simulink model "rov_kinematics_level2"  (R2024b)
settings: Solver=FixedStepAuto  StartTime=0.0  StopTime=90  FixedStep=0.01  RelTol=1e-3
values from neighbouring files (symbols this model uses):
  A = A0    [buildGainGrid.m]    (also in rovHoverModel.m = [ zeros(6),       eye(6))
  B = B0    [buildGainGrid.m]    (also in makeFeedForwardTau.m = p.rho * p.g * p.volume; rovHoverModel.m = [ zeros(6))
  C_integration = C(1:6,:)    [main_hover_controller.m]
  C_real = C_full(meas_idx,:)    [main_hover_controller.m]
  D = diag(p.D_lin) + diag(p.D_quad .* abs(nu))    [computeDynamicsSimple.m]    (also in makeFeedForwardTau.m = D_lin + D_quad; rovHoverModel.m = zeros(12,6))
  Ki = Kfull(:, n+1:end)    [designHoverController.m]    (also in designHoverControllerAtTrim.m)
  L = 0.5    [animateTrajectoryGIF.m]    (also in buildMixingMatrix.m = 0.575; main_hover_controller.m = lqe(A, G, C_real, Qn, Rn); test_linear_hover.m = 400; visualizeTrajectory.m = 1)
undefined symbols (not defined in the file or in its folder): schedData
settings Model: Creator=eirikvarnes  LastModifiedBy=eirikvarnes
settings DataIOCC: SaveFormat=Array  SaveTime=off  ReturnWorkspaceOutputs=off  OutputSaveName=eta

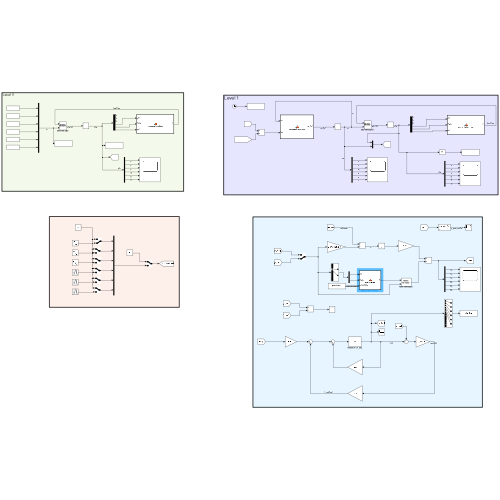
[thumbnail: Simulink's stored preview of the top-level diagram]
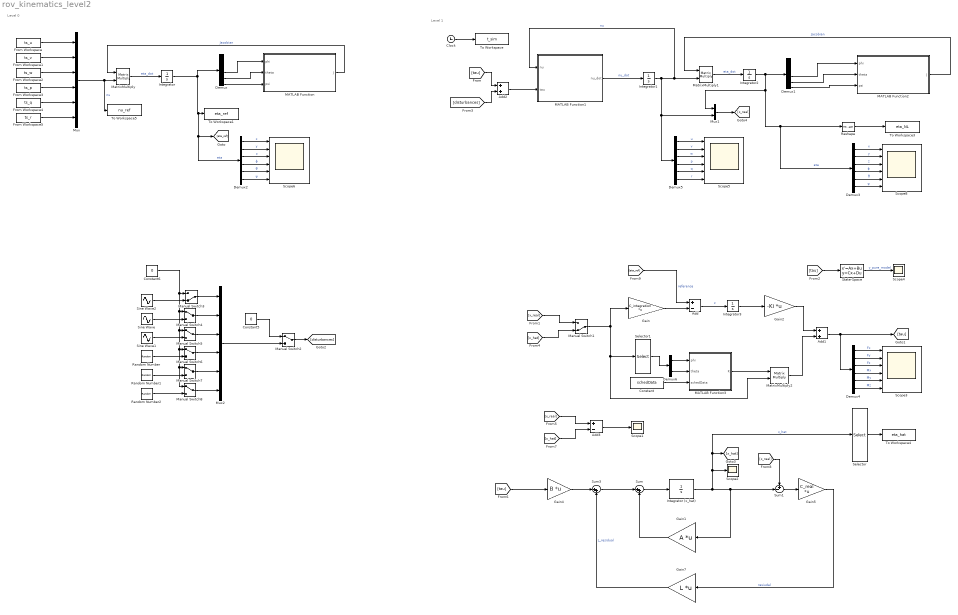
== system rov_kinematics_level2 ==
  note: Level 1
  note: Level 0
  Add : Sum  Inputs=+-
  Add1 : Sum
  Add2 : Sum
  Add3 : Sum  Inputs=+-
  Clock : Clock
  Constant : Constant  Value=schedData  OutDataTypeStr=Bus: schedDataBus
  Constant5 : Constant  Value=0
  Constant6 : Constant  Value=0
  Demux{,1..5} (6 alike) : Demux  Outputs=6
  Demux6 : Demux  Outputs=2
  From Workspace : FromWorkspace  VariableName=ts_u
  From Workspace1 : FromWorkspace  VariableName=ts_v
  From Workspace2 : FromWorkspace  VariableName=ts_w
  From Workspace3 : FromWorkspace  VariableName=ts_p
  From Workspace4 : FromWorkspace  VariableName=ts_q
  From Workspace5 : FromWorkspace  VariableName=ts_r
  Gain : Gain  Gain=C_integration  Multiplication=Matrix(K*u)
  Gain1 : Gain  Gain=A  Multiplication=Matrix(K*u)
  Gain2 : Gain  Gain=-Ki  Multiplication=Matrix(K*u)
  Gain4 : Gain  Gain=B  Multiplication=Matrix(K*u)
  Gain5 : Gain  Gain=C_real  Multiplication=Matrix(K*u)
  Gain7 : Gain  Gain=L  Multiplication=Matrix(K*u)
  Integrator{,1..3} (4 alike) : Integrator
  Integrator (x_hat) : Integrator
  MATLAB Function : MATLAB Function  TreatAsAtomicUnit=on
  MATLAB Function1 : MATLAB Function  TreatAsAtomicUnit=on
  MATLAB Function2 : MATLAB Function  TreatAsAtomicUnit=on
  MATLAB Function3 : MATLAB Function  TreatAsAtomicUnit=on
  Manual Switch1 : ManualSwitch  CurrentSetting=0
  Manual Switch{2,4..8} (6 alike) : ManualSwitch
  Manual Switch3 : ManualSwitch  CurrentSetting=0
  MatrixMultiply : Product  Multiplication=Matrix(*)
  MatrixMultiply1 : Product  Multiplication=Matrix(*)
  MatrixMultiply2 : Product  Multiplication=Matrix(*)
  Mux : Mux  Inputs=6
  Mux1 : Mux  Inputs=2
  Mux2 : Mux  Inputs=6
  Random Number : RandomNumber  Variance=0.01  SampleTime=0.1
  Random Number1 : RandomNumber  Variance=0.01  SampleTime=0.1
  Random Number2 : RandomNumber  Variance=0.01  SampleTime=0.1
  Reshape : Reshape  OutputDimensionality=Customize  OutputDimensions=[6]
  Scope1 : Scope
  Scope2 : Scope
  Scope{3,5..6,8} (4 alike) : Scope  NumInputPorts=6
  Scope4 : Scope
  Selector : Selector  InputPortWidth=12  IndexOptions=Index vector (dialog)  Indices=[1 2 3 4 5 6]  OutputSizes=1
  Selector1 : Selector  InputPortWidth=12  IndexOptions=Index vector (dialog)  Indices=[4 5]  OutputSizes=1
  Sine Wave : Sin  Amplitude=0.1  Frequency=0.05  SampleTime=0
  Sine Wave1 : Sin  Amplitude=0.1  Frequency=0.08  SampleTime=0
  Sine Wave2 : Sin  Amplitude=0.1  Frequency=0.05  SampleTime=0
  State-Space : StateSpace  A=A  B=B  C=eye(12)  D=D  InitialCondition=0
  Sum : Sum  Inputs=|++
  Sum1 : Sum  Inputs=+-|
  Sum3 : Sum  Inputs=|++
  To Workspace : ToWorkspace  VariableName=t_sim  SampleTime=-1
  To Workspace1 : ToWorkspace  VariableName=eta_ref  SampleTime=-1
  To Workspace3 : ToWorkspace  VariableName=eta_NL  SampleTime=-1
  To Workspace4 : ToWorkspace  VariableName=eta_hat  SampleTime=-1
  To Workspace5 : ToWorkspace  VariableName=nu_ref  SampleTime=-1
  wires:
  MATLAB Function1/1(nu_dot) -> Integrator1/1  "nu_dot"
  MATLAB Function2/1(J) -> MatrixMultiply1/1  "Jacobian"
  Demux1/6 -> MATLAB Function2/3(psi)
  Demux1/4 -> MATLAB Function2/1(phi)
  MatrixMultiply1/1 -> Integrator2/1  "eta_dot"
  Demux1/5 -> MATLAB Function2/2(theta)
  Reshape/1 -> To Workspace3/1
  Constant5/1 -> Manual Switch2/1
  Manual Switch3/1 -> Mux2/1
  Sine Wave/1 -> Manual Switch4/2
  Random Number/1 -> Manual Switch6/2
  Manual Switch7/1 -> Mux2/5
  Manual Switch5/1 -> Mux2/3
  Manual Switch4/1 -> Mux2/2
  Manual Switch6/1 -> Mux2/4
  Mux2/1 -> Manual Switch2/2
  Random Number2/1 -> Manual Switch8/2
  Sine Wave2/1 -> Manual Switch3/2
  Manual Switch2/1 -> [disturbances]
  Manual Switch8/1 -> Mux2/6
  Constant6/1 -> Manual Switch8/1, Manual Switch7/1, Manual Switch6/1, Manual Switch5/1, Manual Switch4/1, Manual Switch3/1
  Sine Wave1/1 -> Manual Switch5/2
  Random Number1/1 -> Manual Switch7/2
  Gain2/1 -> Add1/1
  Gain4/1 -> Sum3/1
  State-Space/1 -> Scope4/1  "y_pure_model"
  Integrator3/1 -> Gain2/1
  Demux4/4 -> Scope3/4  "Mx"
  Demux4/1 -> Scope3/1  "Fx"
  [eta_ref] -> Add/1  "reference"
  Add3/1 -> Scope1/1
  Gain5/1 -> Gain7/1  "resiudal"
  Sum1/1 -> Gain5/1
  Integrator (x_hat)/1 -> Selector/1, [x_hat], Scope2/1, Sum1/2, Gain1/1  "x_hat"
  Add/1 -> Integrator3/1  "z"
  Add1/1 -> [tau], Demux4/1
  Gain7/1 -> Sum3/2  "L_residual"
  [x_real] -> Add3/1
  [x_hat] -> Add3/2
  Sum3/1 -> Sum/1
  Sum/1 -> Integrator (x_hat)/1
  Gain1/1 -> Sum/2
  Gain/1 -> Add/2
  MatrixMultiply2/1 -> Add1/2
  [tau] -> Gain4/1
  [x_real] -> Sum1/1
  Demux4/3 -> Scope3/3  "Fz"
  [tau] -> State-Space/1
  [x_real] -> Manual Switch1/1
  [x_hat] -> Manual Switch1/2
  Selector/1 -> To Workspace4/1
  Demux4/2 -> Scope3/2  "Fy"
  Demux4/6 -> Scope3/6  "Mz"
  Demux4/5 -> Scope3/5  "My"
  Integrator2/1 -> Demux1/1, Mux1/1, Demux3/1, Reshape/1  "eta"
  Demux3/1 -> Scope8/1  "x"
  Demux3/5 -> Scope8/5  "θ"
  Demux3/3 -> Scope8/3  "z"
  Demux3/6 -> Scope8/6  "ψ"
  Demux3/4 -> Scope8/4  "ϕ"
  Demux3/2 -> Scope8/2  "y"
  Add2/1 -> MATLAB Function1/2(tau)
  [disturbances] -> Add2/2
  [tau] -> Add2/1
  Demux5/2 -> Scope5/2  "v"
  Demux5/5 -> Scope5/5  "q"
  Demux5/1 -> Scope5/1  "u"
  Demux5/4 -> Scope5/4  "p"
  Demux5/3 -> Scope5/3  "w"
  Demux5/6 -> Scope5/6  "r"
  Integrator1/1 -> Mux1/2, Demux5/1, MATLAB Function1/1(nu), MatrixMultiply1/2  "nu"
  Mux1/1 -> [x_real]
  Clock/1 -> To Workspace/1
  Demux/6 -> MATLAB Function/3(psi)
  MATLAB Function/1(J) -> MatrixMultiply/1  "Jacobian"
  From Workspace2/1 -> Mux/3
  From Workspace5/1 -> Mux/6
  MatrixMultiply/1 -> Integrator/1  "eta_dot"
  From Workspace/1 -> Mux/1
  Demux/4 -> MATLAB Function/1(phi)
  From Workspace1/1 -> Mux/2
  From Workspace3/1 -> Mux/4
  Demux/5 -> MATLAB Function/2(theta)
  From Workspace4/1 -> Mux/5
  Mux/1 -> To Workspace5/1, MatrixMultiply/2  "nu"
  Integrator/1 -> Demux2/1, [eta_ref], To Workspace1/1, Demux/1  "eta"
  Demux2/1 -> Scope6/1  "x"
  Demux2/6 -> Scope6/6  "ψ"
  Demux2/3 -> Scope6/3  "z"
  Demux2/5 -> Scope6/5  "θ"
  Demux2/2 -> Scope6/2  "y"
  Demux2/4 -> Scope6/4  "ϕ"
  Selector1/1 -> Demux6/1
  Demux6/1 -> MATLAB Function3/1(phi)
  Demux6/2 -> MATLAB Function3/2(theta)
  Manual Switch1/1 -> MatrixMultiply2/2, Selector1/1, Gain/1
  Constant/1 -> MATLAB Function3/3(schedData)
  MATLAB Function3/1(K) -> MatrixMultiply2/1

== matlab function rov_kinematics_level2/MATLAB Function1 ==
  data: nu input size=[6 1]; tau input; nu_dot output size=[6 1]
function nu_dot = computeDynamics(nu, tau)
% computeDynamics  1st‐order dynamics with added‐mass & damping only
%   nu_dot = M_R^{-1} * (tau_ff - D*nu)
%
%   Inputs nu and tau_ff must both be 6-by-1 vectors.

  %#codegen
  % Verify inputs are 6-by-1
  assert(all(size(nu)==[6,1]),  'computeDynamics:InvalidInput', 'nu must be 6-by-1');
  assert(all(size(tau)==[6,1]), 'computeDynamics:InvalidInput', 'tau_ff must be 6-by-1');

  % Pull in parameters
  params = rovParameters();

  % Total mass + added‐mass
  M_rb = [params.mass*eye(3), zeros(3);
          zeros(3),           params.I];
  M_A  = -diag([params.Ma_lin; params.Ma_rot]);
  M_R  = M_rb + M_A;

  % Damping
  D_lin  = diag(params.D_lin);
  D_quad = diag(params.D_quad .* abs(nu));
  D      = D_lin + D_quad;

  % Dynamics
  nu_dot = M_R \ (tau - D*nu);
end

== matlab function rov_kinematics_level2/MATLAB Function ==
  data: phi input; J output; theta input; psi input
function J = computeJacobian(phi, theta, psi)
% computeJacobian  ZYX‐Euler Jacobian with singularity clamp
%   Inputs:
%     phi, theta, psi  – Euler angles (roll, pitch, yaw), in radians
%   Output:
%     J  – 6×6 Jacobian mapping [u;v;w;p;q;r] to [xdot;ydot;zdot;phidot;thetadot;psidot]

  %#codegen
  % 1) Rotation matrix R = Rz(psi)*Ry(theta)*Rx(phi)
  cphi = cos(phi);   sphi = sin(phi);
  ctheta = cos(theta); stheta = sin(theta);
  cpsi = cos(psi);   spsi = sin(psi);

  Rz = [ cpsi, -spsi, 0;
         spsi,  cpsi, 0;
           0 ,    0 , 1 ];
  Ry = [ ctheta, 0, stheta;
            0  , 1,   0  ;
        -stheta,0, ctheta ];
  Rx = [ 1,   0  ,   0   ;
         0, cphi, -sphi ;
         0, sphi,  cphi ];
  R = Rz * Ry * Rx;

  % 2) Clamp cos(theta) away from zero to avoid singularity
  epsilon = 5e-3;                          % adjust if needed
  safe_ct = max(abs(ctheta), epsilon) * sign(ctheta);

  % 3) Build T matrix for Euler rates
  %    [phidot; thetadot; psidot] = T * [p; q; r]
  T = [ 1,      sphi*(stheta/safe_ct),   cphi*(stheta/safe_ct);
        0,            cphi,                -sphi;
        0,     sphi/safe_ct,             cphi/safe_ct ];

  % 4) Assemble full Jacobian
  J = [ R,          zeros(3,3);
        zeros(3,3), T       ];
end

== matlab function rov_kinematics_level2/MATLAB Function2 ==
  data: phi input; J output; theta input; psi input
function J = computeJacobian(phi, theta, psi)
% computeJacobian  ZYX‐Euler Jacobian with singularity clamp
%   Inputs:
%     phi, theta, psi  – Euler angles (roll, pitch, yaw), in radians
%   Output:
%     J  – 6×6 Jacobian mapping [u;v;w;p;q;r] to [xdot;ydot;zdot;phidot;thetadot;psidot]

  %#codegen
  % 1) Rotation matrix R = Rz(psi)*Ry(theta)*Rx(phi)
  cphi = cos(phi);   sphi = sin(phi);
  ctheta = cos(theta); stheta = sin(theta);
  cpsi = cos(psi);   spsi = sin(psi);

  Rz = [ cpsi, -spsi, 0;
         spsi,  cpsi, 0;
           0 ,    0 , 1 ];
  Ry = [ ctheta, 0, stheta;
            0  , 1,   0  ;
        -stheta,0, ctheta ];
  Rx = [ 1,   0  ,   0   ;
         0, cphi, -sphi ;
         0, sphi,  cphi ];
  R = Rz * Ry * Rx;

  % 2) Clamp cos(theta) away from zero to avoid singularity
  epsilon = 5e-3;                          % adjust if needed
  safe_ct = max(abs(ctheta), epsilon) * sign(ctheta);

  % 3) Build T matrix for Euler rates
  %    [phidot; thetadot; psidot] = T * [p; q; r]
  T = [ 1,      sphi*(stheta/safe_ct),   cphi*(stheta/safe_ct);
        0,            cphi,                -sphi;
        0,     sphi/safe_ct,             cphi/safe_ct ];

  % 4) Assemble full Jacobian
  J = [ R,          zeros(3,3);
        zeros(3,3), T       ];
end

== matlab function rov_kinematics_level2/MATLAB Function3 ==
  data: phi input; K output; theta input; schedData input
function K = nearestGain(phi, theta, schedData)
%#codegen

    phi_grid   = schedData.phi_grid;
    theta_grid = schedData.theta_grid;
    K_table    = schedData.K_table;

    % Clip phi and theta to the grid bounds
    phi   = min(max(phi, phi_grid(1)),   phi_grid(end));
    theta = min(max(theta, theta_grid(1)), theta_grid(end));

    % Find closest indices
    [~, i] = min(abs(phi_grid - phi));
    [~, j] = min(abs(theta_grid - theta));

    % Lookup gain
    K = K_table(:,:,i,j);
end
